simulink model "invertedPendolum"  (R2019b)
settings: Solver=VariableStepAuto  StartTime=0.0  StopTime=60  FixedStep=0.0001  RelTol=1e-4
InitFcn:
  | simulationVar
values from neighbouring files (symbols this model uses):
  tauMotMax = Ka * Id    (= 6208417600)    [simulationVar.m]
undefined symbols (not defined in the file or in its folder): smiData, X, Y, Z
libraries: sm_lib x29, simulink x6, nesl_utility x3
settings Model: Creator=alfyhack  LastModifiedBy=socci
settings SolverCC: AlgebraicLoopSolver=LineSearch
settings DebuggingCC: UnderSpecifiedDimensionMsg=warning
settings SFSimCC: CustomCodeUndefinedFunction=UseInterfaceOnly

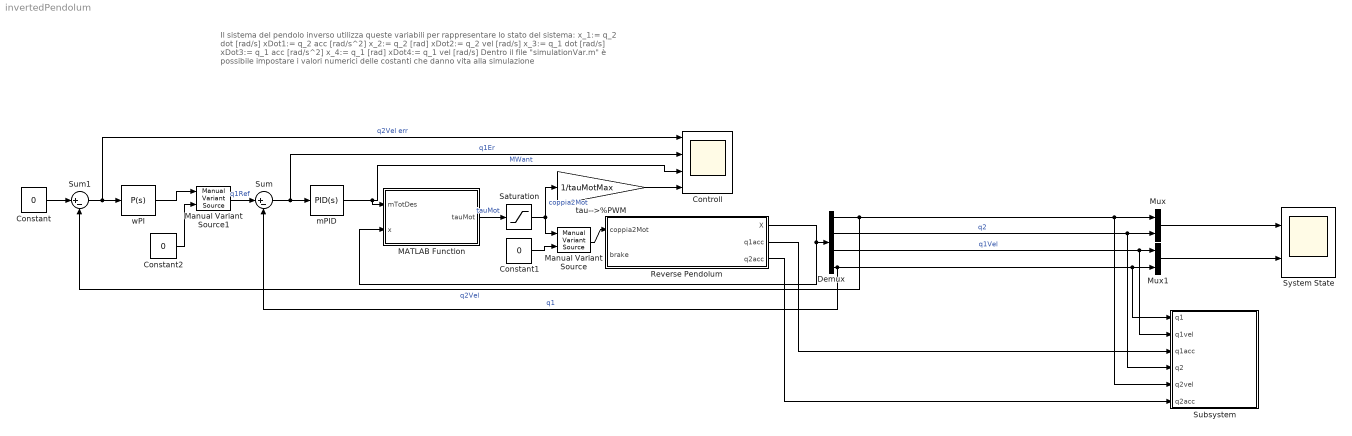
== system invertedPendolum ==
  note: Il sistema del pendolo inverso utilizza queste variabili per rappresentare lo stato del sistema:
      |
      | x_1:= q_2 dot  [rad/s]		xDot1:= q_2 acc   [rad/s^2]
      | x_2:= q_2        [rad]		xDot2:= q_2 vel    [rad/s]
      | x_3:= q_1 dot  [rad/s]		xDot3:= q_1 acc   [rad/s^2]
      | x_4:= q_1        [rad]		xDot4:= q_1 vel    [rad/s]
      |
      | Dentro il file "simulationVar.m" è possibile impostare i valori numerici delle costanti che danno vita alla simulazione
  Constant : Constant  Value=0
  Constant1 : Constant  Value=0
  Constant2 : Constant  Value=0
  Controll : Scope  NumInputPorts=4
  Demux : Demux
  MATLAB Function : MATLAB Function  TreatAsAtomicUnit=on
  Manual Variant Source : simulink/Signal Routing/Manual Variant Source  NumChoices=2  LabelModeActiveChoice=V_1
      settings: SourceProductName=Simulink
  Manual Variant Source1 : simulink/Signal Routing/Manual Variant Source  NumChoices=2  LabelModeActiveChoice=V_1
      settings: SourceProductName=Simulink
  Mux : Mux  Inputs=2
  Mux1 : Mux  Inputs=2
  Reverse Pendolum : Subsystem
  Saturation : Saturate  UpperLimit=tauMotMax  LowerLimit=-tauMotMax
  Subsystem : Subsystem
  Sum : Sum  Inputs=|+-
  Sum1 : Sum  Inputs=|+-
  System State : Scope  NumInputPorts=2
  mPID : simulink/Continuous/PID Controller  Controller=PID  Form=Parallel  TimeDomain=Continuous-time  SampleTime=-1  IntegratorMethod=Forward Euler  FilterMethod=Forward Euler  ControllerParametersSource=internal  P=44059890.2523914  I=6444277.98639226  D=74154463.3015082  UseFilter=on  N=34.9657186034109  TunerSelectOption=Transfer Function Based (PID Tuner App)  InitialConditionSource=internal  InitialConditionForIntegrator=0  InitialConditionForFilter=0  DifferentiatorICPrevScaledInput=0  ExternalReset=none  TrackingMode=off  Kt=1  LimitOutput=off  UpperSaturationLimit=1000  LowerSaturationLimit=1000  LinearizeAsGain=off  AntiWindupMode=none  Kb=1  POutMin=[]  POutMax=[]  IOutMin=[]  IOutMax=[]  DOutMin=[]  DOutMax=[]  NOutMin=[]  NOutMax=[]  SumOutMin=[]  SumOutMax=[]  SaturationOutMin=[]  SaturationOutMax=[]  PParamMin=[]  PParamMax=[]  IParamMin=[]  IParamMax=[]  DParamMin=[]  DParamMax=[]  NParamMin=[]  NParamMax=[]  KbParamMin=[]  KbParamMax=[]  KtParamMin=[]  KtParamMax=[]  KbOutMin=[]  KbOutMax=[]  KtOutMin=[]  KtOutMax=[]  IntegratorOutMin=[]  IntegratorOutMax=[]  FilterOutMin=[]  FilterOutMax=[]  SumI1OutMin=[]  SumI1OutMax=[]  SumI2OutMin=[]  SumI2OutMax=[]  SumI3OutMin=[]  SumI3OutMax=[]  SumI4OutMin=[]  SumI4OutMax=[]  SumDOutMin=[]  SumDOutMax=[]  DifferentiatorOutMin=[]  DifferentiatorOutMax=[]  FilterDiffOutCoefMin=[]  FilterDiffOutCoefMax=[]  ReciprocalOutMin=[]  ReciprocalOutMax=[]  SumDenOutMin=[]  SumDenOutMax=[]  SumNumOutMin=[]  SumNumOutMax=[]  DivideOutMin=[]  DivideOutMax=[]  IntegratorContinuousStateAttributes=''  IntegratorStateMustResolveToSignalObject=off  IntegratorRTWStateStorageClass=Auto  FilterContinuousStateAttributes=''  FilterStateMustResolveToSignalObject=off  FilterRTWStateStorageClass=Auto  ParallelPVariant=InternalParameters  IdealPVariant=Disabled  IVariant=InternalParameters  DVariant=InternalParameters  IntegratorVariant=Continuous  SatVariant=Disabled  AWVariant=Passthrough  PCopyVariant=Disabled  TRVariant=Disabled  FdbkBlocksVariant=Forward  IdealPFdbkVariant=Disabled  SatFdbkVariant=Disabled  DerivativeFilterVariant=ContFilter  NVariant=InternalParameters  NCopyVariant=Disabled  FilterICVariant=InternalICsFilter  IntegratorICVariant=InternalICs  ExternalResetVariant=Disabled  TRSumVariant=Passthrough  SumFdbkVariant=Disabled  SumVariant=Sum_PID
  tau-->%PWM : Gain  Gain=1/tauMotMax
  wPI : simulink/Continuous/PID Controller  Controller=P  Form=Parallel  TimeDomain=Continuous-time  SampleTime=-1  IntegratorMethod=Forward Euler  FilterMethod=Forward Euler  ControllerParametersSource=internal  P=0.000273498312206375  I=0.001  D=1  UseFilter=on  N=2000  TunerSelectOption=Transfer Function Based (PID Tuner App)  InitialConditionSource=internal  InitialConditionForIntegrator=0  InitialConditionForFilter=0  DifferentiatorICPrevScaledInput=0  ExternalReset=none  TrackingMode=off  Kt=1  LimitOutput=on  UpperSaturationLimit=0.1  LowerSaturationLimit=-0.1  LinearizeAsGain=off  AntiWindupMode=none  Kb=1  POutMin=[]  POutMax=[]  IOutMin=[]  IOutMax=[]  DOutMin=[]  DOutMax=[]  NOutMin=[]  NOutMax=[]  SumOutMin=[]  SumOutMax=[]  SaturationOutMin=[]  SaturationOutMax=[]  PParamMin=[]  PParamMax=[]  IParamMin=[]  IParamMax=[]  DParamMin=[]  DParamMax=[]  NParamMin=[]  NParamMax=[]  KbParamMin=[]  KbParamMax=[]  KtParamMin=[]  KtParamMax=[]  KbOutMin=[]  KbOutMax=[]  KtOutMin=[]  KtOutMax=[]  IntegratorOutMin=[]  IntegratorOutMax=[]  FilterOutMin=[]  FilterOutMax=[]  SumI1OutMin=[]  SumI1OutMax=[]  SumI2OutMin=[]  SumI2OutMax=[]  SumI3OutMin=[]  SumI3OutMax=[]  SumI4OutMin=[]  SumI4OutMax=[]  SumDOutMin=[]  SumDOutMax=[]  DifferentiatorOutMin=[]  DifferentiatorOutMax=[]  FilterDiffOutCoefMin=[]  FilterDiffOutCoefMax=[]  ReciprocalOutMin=[]  ReciprocalOutMax=[]  SumDenOutMin=[]  SumDenOutMax=[]  SumNumOutMin=[]  SumNumOutMax=[]  DivideOutMin=[]  DivideOutMax=[]  IntegratorContinuousStateAttributes=''  IntegratorStateMustResolveToSignalObject=off  IntegratorRTWStateStorageClass=Auto  FilterContinuousStateAttributes=''  FilterStateMustResolveToSignalObject=off  FilterRTWStateStorageClass=Auto  ParallelPVariant=InternalParameters  IdealPVariant=Disabled  IVariant=Disabled  DVariant=Disabled  IntegratorVariant=Disabled  SatVariant=Enabled  AWVariant=Disabled  PCopyVariant=Disabled  TRVariant=Disabled  FdbkBlocksVariant=Forward  IdealPFdbkVariant=Disabled  SatFdbkVariant=Disabled  DerivativeFilterVariant=Disabled  NVariant=Disabled  NCopyVariant=Disabled_SignalSpec  FilterICVariant=Disabled  IntegratorICVariant=Disabled  ExternalResetVariant=Disabled  TRSumVariant=Passthrough  SumFdbkVariant=Disabled  SumVariant=Passthrough_P
  wires:
  Demux/4 -> Subsystem/1(q1), Mux1/2, Sum/2  "q1"
  Demux/1 -> Subsystem/5(q2vel), Mux/1, Sum1/2  "q2Vel"
  MATLAB Function/1(tauMot) -> Saturation/1  "tauMot"
  mPID/1 -> Controll/3, MATLAB Function/1(mTotDes)  "MWant"
  Sum/1 -> Controll/2, mPID/1  "q1Er"
  wPI/1 -> Manual Variant Source1/1
  Constant/1 -> Sum1/1
  Sum1/1 -> Controll/1, wPI/1  "q2Vel err"
  Saturation/1 -> tau-->%PWM/1, Manual Variant Source/1  "coppia2Mot"
  Reverse Pendolum/1(X) -> Demux/1, MATLAB Function/2(x)
  Demux/3 -> Subsystem/2(q1vel), Mux1/1  "q1Vel"
  Mux1/1 -> System State/2
  Mux/1 -> System State/1
  tau-->%PWM/1 -> Controll/4
  Manual Variant Source/1 -> Reverse Pendolum/1(coppia2Mot)
  Constant1/1 -> Manual Variant Source/2
  Manual Variant Source1/1 -> Sum/1  "q1Ref"
  Constant2/1 -> Manual Variant Source1/2
  Reverse Pendolum/2(q1acc) -> Subsystem/3(q1acc)
  Reverse Pendolum/3(q2acc) -> Subsystem/6(q2acc)
  Demux/2 -> Subsystem/4(q2), Mux/2  "q2"

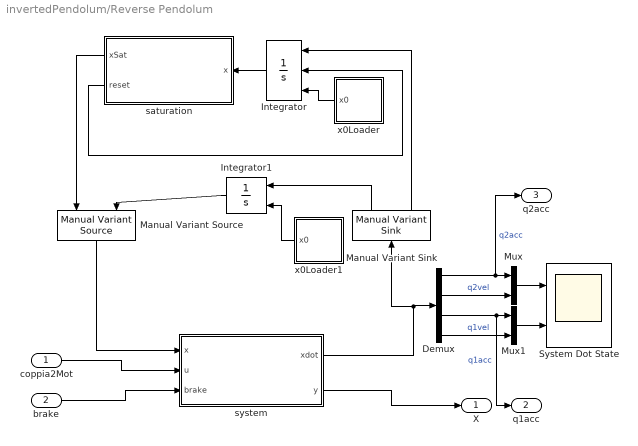
== system invertedPendolum/Reverse Pendolum ==
  coppia2Mot : Inport
  brake : Inport  Port=2
  Demux : Demux
  Integrator : Integrator  ExternalReset=rising  InitialConditionSource=external  InitialCondition=[0,0.1,0]
  Integrator1 : Integrator  InitialConditionSource=external
  Manual Variant Sink : simulink/Signal Routing/Manual Variant Sink  NumChoices=2  LabelModeActiveChoice=V_2
      settings: SourceProductName=Simulink
  Manual Variant Source : simulink/Signal Routing/Manual Variant Source  NumChoices=2  LabelModeActiveChoice=V_1
      settings: SourceProductName=Simulink
  Mux : Mux  Inputs=2
  Mux1 : Mux  Inputs=2
  System Dot State : Scope  NumInputPorts=2
  saturation : MATLAB Function  TreatAsAtomicUnit=on
  system : MATLAB Function  TreatAsAtomicUnit=on
  x0Loader : MATLAB Function  TreatAsAtomicUnit=on
  x0Loader1 : MATLAB Function  TreatAsAtomicUnit=on
  X : Outport  VectorParamsAs1DForOutWhenUnconnected=off
  q1acc : Outport  Port=2  VectorParamsAs1DForOutWhenUnconnected=off
  q2acc : Outport  Port=3  VectorParamsAs1DForOutWhenUnconnected=off
  wires:
  x0Loader/1(x0) -> Integrator/3
  Integrator/1 -> saturation/1(x)
  saturation/2(reset) -> Integrator/2
  coppia2Mot/1 -> system/2(u)
  system/2(y) -> X/1
  Mux/1 -> System Dot State/1
  Demux/3 -> q1acc/1, Mux1/1  "q1acc"
  Demux/1 -> q2acc/1, Mux/1  "q2acc"
  system/1(xdot) -> Manual Variant Sink/1, Demux/1
  Demux/2 -> Mux/2  "q2vel"
  Demux/4 -> Mux1/2  "q1vel"
  Mux1/1 -> System Dot State/2
  Manual Variant Sink/2 -> Integrator/1
  saturation/1(xSat) -> Manual Variant Source/1
  Integrator1/1 -> Manual Variant Source/2
  Manual Variant Sink/1 -> Integrator1/1
  Manual Variant Source/1 -> system/1(x)
  x0Loader1/1(x0) -> Integrator1/2
  brake/1 -> system/3(brake)

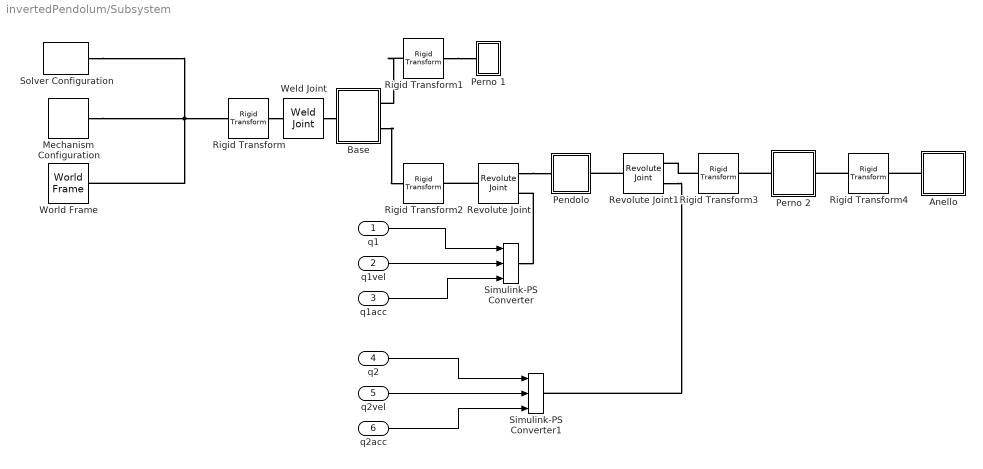
== system invertedPendolum/Subsystem ==
  q1 : Inport
  q1vel : Inport  Port=2
  q1acc : Inport  Port=3
  q2 : Inport  Port=4
  q2vel : Inport  Port=5
  q2acc : Inport  Port=6
  "Anello " : Subsystem
  Base : Subsystem
  Mechanism Configuration : sm_lib/Utilities/Mechanism Configuration  UniformGravity=Constant  GravityVector=[0 0 0]  GravityUnits=m/s^2  LinearizationDelta=0.001
  Pendolo : Subsystem
  Perno 1 : Subsystem
  Perno 2 : Subsystem
  Revolute Joint : sm_lib/Joints/Revolute Joint  JointMode=Normal  SenseConstraintForce=off  SenseConstraintForceX=off  SenseConstraintForceY=off  SenseConstraintForceZ=off  SenseConstraintTorque=off  SenseConstraintTorqueX=off  SenseConstraintTorqueY=off  SenseConstraintTorqueZ=off  SenseTotalForce=off  SenseTotalForceX=off  SenseTotalForceY=off  SenseTotalForceZ=off  SenseTotalTorque=off  SenseTotalTorqueX=off  SenseTotalTorqueY=off  SenseTotalTorqueZ=off  CompositeWrenchDir=FollowerOnBase  CompositeWrenchFrame=BaseFrame  EquilibriumPosition=0  EquilibriumPositionUnits=deg  SpringStiffness=0  SpringStiffnessUnits=N*m/deg  DampingCoefficient=0  DampingCoefficientUnits=N*m/(deg/s)  TorqueActuationMode=ComputedTorque  MotionActuationMode=InputMotion  SensePosition=off  SenseVelocity=off  SenseAcceleration=off  SenseTorqueForce=off  SenseLowerLimitTorqueForce=off  SenseUpperLimitTorqueForce=off  LowerLimitSpecify=off  LowerLimitBound=-90  LowerLimitBoundUnits=deg  LowerLimitStiffness=1e4  LowerLimitStiffnessUnits=N*m/deg  LowerLimitDamping=10  LowerLimitDampingUnits=N*m/(deg/s)  LowerLimitTransitionRegionWidth=0.1  LowerLimitTransitionRegionWidthUnits=deg  UpperLimitSpecify=off  UpperLimitBound=90  UpperLimitBoundUnits=deg  UpperLimitStiffness=1e4  UpperLimitStiffnessUnits=N*m/deg  UpperLimitDamping=10  UpperLimitDampingUnits=N*m/(deg/s)  UpperLimitTransitionRegionWidth=0.1  UpperLimitTransitionRegionWidthUnits=deg  PositionTargetSpecify=on  PositionTargetPriority=Low  PositionTargetValue=smiData.RevoluteJoint(2).Rz.Pos  PositionTargetValueUnits=deg  VelocityTargetSpecify=off  VelocityTargetPriority=High  VelocityTargetValue=0  VelocityTargetValueUnits=deg/s
  Revolute Joint1 : sm_lib/Joints/Revolute Joint  JointMode=Normal  SenseConstraintForce=off  SenseConstraintForceX=off  SenseConstraintForceY=off  SenseConstraintForceZ=off  SenseConstraintTorque=off  SenseConstraintTorqueX=off  SenseConstraintTorqueY=off  SenseConstraintTorqueZ=off  SenseTotalForce=off  SenseTotalForceX=off  SenseTotalForceY=off  SenseTotalForceZ=off  SenseTotalTorque=off  SenseTotalTorqueX=off  SenseTotalTorqueY=off  SenseTotalTorqueZ=off  CompositeWrenchDir=FollowerOnBase  CompositeWrenchFrame=BaseFrame  EquilibriumPosition=0  EquilibriumPositionUnits=deg  SpringStiffness=0  SpringStiffnessUnits=N*m/deg  DampingCoefficient=0  DampingCoefficientUnits=N*m/(deg/s)  TorqueActuationMode=ComputedTorque  MotionActuationMode=InputMotion  SensePosition=off  SenseVelocity=off  SenseAcceleration=off  SenseTorqueForce=off  SenseLowerLimitTorqueForce=off  SenseUpperLimitTorqueForce=off  LowerLimitSpecify=off  LowerLimitBound=-90  LowerLimitBoundUnits=deg  LowerLimitStiffness=1e4  LowerLimitStiffnessUnits=N*m/deg  LowerLimitDamping=10  LowerLimitDampingUnits=N*m/(deg/s)  LowerLimitTransitionRegionWidth=0.1  LowerLimitTransitionRegionWidthUnits=deg  UpperLimitSpecify=off  UpperLimitBound=90  UpperLimitBoundUnits=deg  UpperLimitStiffness=1e4  UpperLimitStiffnessUnits=N*m/deg  UpperLimitDamping=10  UpperLimitDampingUnits=N*m/(deg/s)  UpperLimitTransitionRegionWidth=0.1  UpperLimitTransitionRegionWidthUnits=deg  PositionTargetSpecify=off  PositionTargetPriority=High  PositionTargetValue=0  PositionTargetValueUnits=deg  VelocityTargetSpecify=off  VelocityTargetPriority=High  VelocityTargetValue=0  VelocityTargetValueUnits=deg/s
  Rigid Transform{,1,3..4} (4 alike) : sm_lib/Frames and Transforms/Rigid Transform  TranslationMethod=None  TranslationStandardOffset=0  TranslationLengthUnit=m  TranslationStandardAxis=+Z  TranslationCartesianOffset=[0 0 0]  TranslationROffset=0  TranslationROffsetUnits=m  TranslationZOffset=0  TranslationZOffsetUnits=m  TranslationThetaOffset=0  TranslationThetaOffsetUnits=deg  RotationMethod=None  RotationAngleUnits=deg  RotationStandardAxis=+Z  RotationAngle=0.0  RotationArbitraryAxis=[0 0 1]  FollAlignAxisA=+X  BaseAlignAxisA=+Y  FollAlignAxisB=+Y  BaseAlignAxisB=+Z  RotationSequenceAxes=FollowerAxes  RotationSequence=XYX  RotationSequenceAngles=[0 0 0]  RotationSequenceAnglesUnits=deg  RotationMatrix=[1 0 0; 0 1 0; 0 0 1]
  Rigid Transform2 : sm_lib/Frames and Transforms/Rigid Transform  TranslationMethod=None  TranslationStandardOffset=0  TranslationLengthUnit=m  TranslationStandardAxis=+Z  TranslationCartesianOffset=[0 0 0]  TranslationROffset=0  TranslationROffsetUnits=m  TranslationZOffset=0  TranslationZOffsetUnits=m  TranslationThetaOffset=0  TranslationThetaOffsetUnits=deg  RotationMethod=RotationSequence  RotationAngleUnits=deg  RotationStandardAxis=+Z  RotationAngle=0.0  RotationArbitraryAxis=[0 0 1]  FollAlignAxisA=+X  BaseAlignAxisA=+Y  FollAlignAxisB=+Y  BaseAlignAxisB=+Z  RotationSequenceAxes=FollowerAxes  RotationSequence=XYZ  RotationSequenceAngles=[0 0 90 ]  RotationSequenceAnglesUnits=deg  RotationMatrix=[1 0 0; 0 1 0; 0 0 1]
  Simulink-PS Converter : nesl_utility/Simulink-PS Converter  PhysicalDomain=network_engine_domain  SubClassName=ps_input  LeftPortType=input  RightPortType=output  PseudoPeriodic=off  Frequencies=[]  NoiseDistribution=none  NoiseParameters=[]  Unit=1  AffineConversion=off  FilteringAndDerivatives=provide  SimscapeFilterOrder=1  InputFilterTimeConstant=0.001  UdotUserProvided=2
  Simulink-PS Converter1 : nesl_utility/Simulink-PS Converter  PhysicalDomain=network_engine_domain  SubClassName=ps_input  LeftPortType=input  RightPortType=output  PseudoPeriodic=off  Frequencies=[]  NoiseDistribution=none  NoiseParameters=[]  Unit=1  AffineConversion=off  FilteringAndDerivatives=provide  SimscapeFilterOrder=1  InputFilterTimeConstant=0.001  UdotUserProvided=2
  Solver Configuration : nesl_utility/Solver Configuration  PhysicalDomain=network_engine_domain  SubClassName=solver  LeftPortType=input  RightPortType=generic  Tones=[]  Harmonics=[]  SimulateNoise=off  Profile=off  UseLocalSampling=off  EnableSwitchedLinearOptims=on  FrequencyDomain=off  UseCCode=off  RelTol=0.001  AbsTol=1e-06  MinStep=1e-09  ToWorkspace=off  RevertToSquareIcSolve=off  NumHomotopyIterations=100  PhasorMode=off  PhasorModeNumHarmonics=1  DoDC=off  ResidualTolerance=1e-09  UseLocalSolver=off  LocalSolverChoice=NE_BACKWARD_EULER_ADVANCER  LocalSolverSampleTime=0.001  DoFixedCost=off  MaxNonlinIter=3  MaxModeIter=2  LinearAlgebra=auto  EquationFormulation=NE_TIME_EF  DelaysMemoryBudget=1024  AutomaticFiltering=on  FilteringTimeConstant=0.001  PartitionStorageMethod=AS_NEEDED  PartitionMemoryBudget=1024  PartitionMethod=ROBUST
  Weld Joint : sm_lib/Joints/Weld Joint  JointMode=Normal  SenseConstraintForce=off  SenseConstraintForceX=off  SenseConstraintForceY=off  SenseConstraintForceZ=off  SenseConstraintTorque=off  SenseConstraintTorqueX=off  SenseConstraintTorqueY=off  SenseConstraintTorqueZ=off  SenseTotalForce=off  SenseTotalForceX=off  SenseTotalForceY=off  SenseTotalForceZ=off  SenseTotalTorque=off  SenseTotalTorqueX=off  SenseTotalTorqueY=off  SenseTotalTorqueZ=off  CompositeWrenchDir=FollowerOnBase  CompositeWrenchFrame=BaseFrame
  World Frame : sm_lib/Frames and Transforms/World Frame
  wires:
  q1/1 -> Simulink-PS Converter/1
  q1vel/1 -> Simulink-PS Converter/2
  q1acc/1 -> Simulink-PS Converter/3
  q2acc/1 -> Simulink-PS Converter1/3
  q2/1 -> Simulink-PS Converter1/1
  q2vel/1 -> Simulink-PS Converter1/2
  connections:
  Solver Configuration/RConn1 -- World Frame/RConn1 -- Rigid Transform/LConn1 -- Mechanism Configuration/RConn1
  Rigid Transform/RConn1 -- Weld Joint/LConn1
  Weld Joint/RConn1 -- Base/LConn1
  Rigid Transform1/LConn1 -- Base/RConn1
  Rigid Transform1/RConn1 -- Perno 1/LConn1
  Base/RConn2 -- Rigid Transform2/LConn1
  Revolute Joint/RConn1 -- Rigid Transform2/RConn1
  Simulink-PS Converter/RConn1 -- Revolute Joint/LConn2
  Revolute Joint/LConn1 -- Pendolo/LConn1
  Revolute Joint1/RConn1 -- Pendolo/RConn1
  Rigid Transform3/RConn1 -- Revolute Joint1/LConn1
  Perno 2/LConn1 -- Rigid Transform3/LConn1
  Rigid Transform4/LConn1 -- Perno 2/RConn1
  "Anello "/LConn1 -- Rigid Transform4/RConn1
  Revolute Joint1/LConn2 -- Simulink-PS Converter1/RConn1

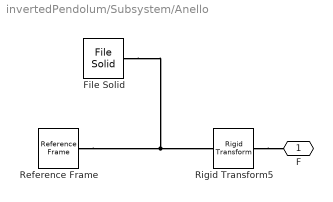
== system invertedPendolum/Subsystem/Anello  ==
  File Solid : sm_lib/Body Elements/File Solid  ExtGeomFileName=Anello_ipt_98140efb.STEP  UnitType=FromFile  ExtGeomFileUnits=m  StepReaderType=HEX  ExportEntireGeometry=off  InertiaType=Custom  Mass=smiData.Solid(4).mass  MassUnits=kg  CenterOfMass=smiData.Solid(4).CoM  CenterOfMassUnits=mm  MomentsOfInertia=smiData.Solid(4).MoI  MomentsOfInertiaUnits=kg*mm^2  ProductsOfInertia=smiData.Solid(4).PoI  ProductsOfInertiaUnits=kg*mm^2  BasedOnType=DensityFromFile  Density=1000  DensityUnits=kg/m^3  DoExposeReferenceFrame=on  SerializedFrames=<Frames/>  GraphicType=FromGeometry  MarkerShape=Sphere  MarkerSize=10  GraphicVisPropType=SimpleVisualProperties  GraphicDiffuseColor=[0.8 1.0 0.2]  GraphicSpecularColor=[0.5 0.5 0.5 1.0]  GraphicAmbientColor=[0.15 0.15 0.15 1.0]  GraphicEmissiveColor=[0.0 0.0 0.0 1.0]  GraphicShininess=75  GraphicOpacity=1.0
  Reference Frame : sm_lib/Frames and Transforms/Reference Frame
  Rigid Transform5 : sm_lib/Frames and Transforms/Rigid Transform  TranslationMethod=Cartesian  TranslationStandardOffset=0  TranslationLengthUnit=mm  TranslationStandardAxis=+Z  TranslationCartesianOffset=smiData.RigidTransform(9).translation  TranslationROffset=0  TranslationROffsetUnits=m  TranslationZOffset=0  TranslationZOffsetUnits=m  TranslationThetaOffset=0  TranslationThetaOffsetUnits=deg  RotationMethod=ArbitraryAxis  RotationAngleUnits=rad  RotationStandardAxis=+Z  RotationAngle=smiData.RigidTransform(9).angle  RotationArbitraryAxis=smiData.RigidTransform(9).axis  FollAlignAxisA=+X  BaseAlignAxisA=+Y  FollAlignAxisB=+Y  BaseAlignAxisB=+Z  RotationSequenceAxes=FollowerAxes  RotationSequence=XYX  RotationSequenceAngles=[0 0 0]  RotationSequenceAnglesUnits=deg  RotationMatrix=[1 0 0; 0 1 0; 0 0 1]
  F : PMIOPort  Side=Left
  connections:
  Reference Frame/RConn1 -- File Solid/RConn1 -- Rigid Transform5/LConn1
  Rigid Transform5/RConn1 -- F/RConn1

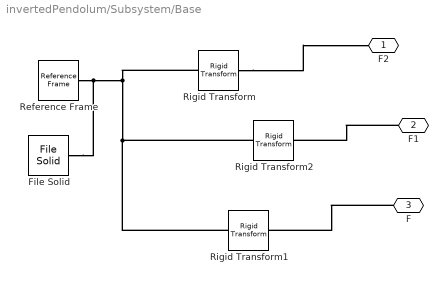
== system invertedPendolum/Subsystem/Base ==
  File Solid : sm_lib/Body Elements/File Solid  ExtGeomFileName=Base_ipt_2f93e7fb.STEP  UnitType=FromFile  ExtGeomFileUnits=m  StepReaderType=HEX  ExportEntireGeometry=off  InertiaType=Custom  Mass=smiData.Solid(1).mass  MassUnits=kg  CenterOfMass=smiData.Solid(1).CoM  CenterOfMassUnits=mm  MomentsOfInertia=smiData.Solid(1).MoI  MomentsOfInertiaUnits=kg*mm^2  ProductsOfInertia=smiData.Solid(1).PoI  ProductsOfInertiaUnits=kg*mm^2  BasedOnType=DensityFromFile  Density=1000  DensityUnits=kg/m^3  DoExposeReferenceFrame=on  SerializedFrames=<Frames/>  GraphicType=FromGeometry  MarkerShape=Sphere  MarkerSize=10  GraphicVisPropType=SimpleVisualProperties  GraphicDiffuseColor=[0.2 0.2 1.0]  GraphicSpecularColor=[0.5 0.5 0.5 1.0]  GraphicAmbientColor=[0.15 0.15 0.15 1.0]  GraphicEmissiveColor=[0.0 0.0 0.0 1.0]  GraphicShininess=75  GraphicOpacity=1.0
  Reference Frame : sm_lib/Frames and Transforms/Reference Frame
  Rigid Transform : sm_lib/Frames and Transforms/Rigid Transform  TranslationMethod=Cartesian  TranslationStandardOffset=0  TranslationLengthUnit=mm  TranslationStandardAxis=+Z  TranslationCartesianOffset=smiData.RigidTransform(6).translation  TranslationROffset=0  TranslationROffsetUnits=m  TranslationZOffset=0  TranslationZOffsetUnits=m  TranslationThetaOffset=0  TranslationThetaOffsetUnits=deg  RotationMethod=ArbitraryAxis  RotationAngleUnits=rad  RotationStandardAxis=+Z  RotationAngle=smiData.RigidTransform(6).angle  RotationArbitraryAxis=smiData.RigidTransform(6).axis  FollAlignAxisA=+X  BaseAlignAxisA=+Y  FollAlignAxisB=+Y  BaseAlignAxisB=+Z  RotationSequenceAxes=FollowerAxes  RotationSequence=XYX  RotationSequenceAngles=[0 0 0]  RotationSequenceAnglesUnits=deg  RotationMatrix=[1 0 0; 0 1 0; 0 0 1]
  Rigid Transform1 : sm_lib/Frames and Transforms/Rigid Transform  TranslationMethod=Cartesian  TranslationStandardOffset=0  TranslationLengthUnit=mm  TranslationStandardAxis=+Z  TranslationCartesianOffset=smiData.RigidTransform(1).translation  TranslationROffset=0  TranslationROffsetUnits=m  TranslationZOffset=0  TranslationZOffsetUnits=m  TranslationThetaOffset=0  TranslationThetaOffsetUnits=deg  RotationMethod=ArbitraryAxis  RotationAngleUnits=rad  RotationStandardAxis=+Z  RotationAngle=smiData.RigidTransform(1).angle  RotationArbitraryAxis=smiData.RigidTransform(1).axis  FollAlignAxisA=+X  BaseAlignAxisA=+Y  FollAlignAxisB=+Y  BaseAlignAxisB=+Z  RotationSequenceAxes=FollowerAxes  RotationSequence=XYX  RotationSequenceAngles=[0 0 0]  RotationSequenceAnglesUnits=deg  RotationMatrix=[1 0 0; 0 1 0; 0 0 1]
  Rigid Transform2 : sm_lib/Frames and Transforms/Rigid Transform  TranslationMethod=Cartesian  TranslationStandardOffset=0  TranslationLengthUnit=mm  TranslationStandardAxis=+Z  TranslationCartesianOffset=smiData.RigidTransform(4).translation  TranslationROffset=0  TranslationROffsetUnits=m  TranslationZOffset=0  TranslationZOffsetUnits=m  TranslationThetaOffset=0  TranslationThetaOffsetUnits=deg  RotationMethod=ArbitraryAxis  RotationAngleUnits=rad  RotationStandardAxis=+Z  RotationAngle=smiData.RigidTransform(4).angle  RotationArbitraryAxis=smiData.RigidTransform(4).axis  FollAlignAxisA=+X  BaseAlignAxisA=+Y  FollAlignAxisB=+Y  BaseAlignAxisB=+Z  RotationSequenceAxes=FollowerAxes  RotationSequence=XYX  RotationSequenceAngles=[0 0 0]  RotationSequenceAnglesUnits=deg  RotationMatrix=[1 0 0; 0 1 0; 0 0 1]
  F2 : PMIOPort  Side=Right
  F1 : PMIOPort  Port=2  Side=Right
  F : PMIOPort  Port=3  Side=Left
  connections:
  Reference Frame/RConn1 -- File Solid/RConn1 -- Rigid Transform1/LConn1 -- Rigid Transform2/LConn1 -- Rigid Transform/LConn1
  Rigid Transform/RConn1 -- F2/RConn1
  F1/RConn1 -- Rigid Transform2/RConn1
  F/RConn1 -- Rigid Transform1/RConn1

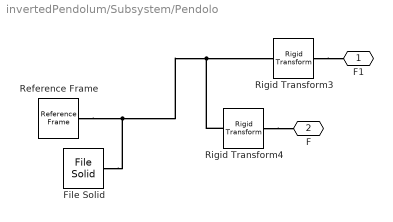
== system invertedPendolum/Subsystem/Pendolo ==
  File Solid : sm_lib/Body Elements/File Solid  ExtGeomFileName=Pendolo_ipt_9bec4f24.STEP  UnitType=FromFile  ExtGeomFileUnits=m  StepReaderType=HEX  ExportEntireGeometry=off  InertiaType=Custom  Mass=smiData.Solid(3).mass  MassUnits=kg  CenterOfMass=smiData.Solid(3).CoM  CenterOfMassUnits=mm  MomentsOfInertia=smiData.Solid(3).MoI  MomentsOfInertiaUnits=kg*mm^2  ProductsOfInertia=smiData.Solid(3).PoI  ProductsOfInertiaUnits=kg*mm^2  BasedOnType=DensityFromFile  Density=1000  DensityUnits=kg/m^3  DoExposeReferenceFrame=on  SerializedFrames=<Frames/>  GraphicType=FromGeometry  MarkerShape=Sphere  MarkerSize=10  GraphicVisPropType=SimpleVisualProperties  GraphicDiffuseColor=[0.8 1.0 0.2]  GraphicSpecularColor=[0.5 0.5 0.5 1.0]  GraphicAmbientColor=[0.15 0.15 0.15 1.0]  GraphicEmissiveColor=[0.0 0.0 0.0 1.0]  GraphicShininess=75  GraphicOpacity=1.0
  Reference Frame : sm_lib/Frames and Transforms/Reference Frame
  Rigid Transform3 : sm_lib/Frames and Transforms/Rigid Transform  TranslationMethod=Cartesian  TranslationStandardOffset=0  TranslationLengthUnit=mm  TranslationStandardAxis=+Z  TranslationCartesianOffset=smiData.RigidTransform(8).translation  TranslationROffset=0  TranslationROffsetUnits=m  TranslationZOffset=0  TranslationZOffsetUnits=m  TranslationThetaOffset=0  TranslationThetaOffsetUnits=deg  RotationMethod=ArbitraryAxis  RotationAngleUnits=rad  RotationStandardAxis=+Z  RotationAngle=smiData.RigidTransform(8).angle  RotationArbitraryAxis=smiData.RigidTransform(8).axis  FollAlignAxisA=+X  BaseAlignAxisA=+Y  FollAlignAxisB=+Y  BaseAlignAxisB=+Z  RotationSequenceAxes=FollowerAxes  RotationSequence=XYX  RotationSequenceAngles=[0 0 0]  RotationSequenceAnglesUnits=deg  RotationMatrix=[1 0 0; 0 1 0; 0 0 1]
  Rigid Transform4 : sm_lib/Frames and Transforms/Rigid Transform  TranslationMethod=Cartesian  TranslationStandardOffset=0  TranslationLengthUnit=mm  TranslationStandardAxis=+Z  TranslationCartesianOffset=smiData.RigidTransform(3).translation  TranslationROffset=0  TranslationROffsetUnits=m  TranslationZOffset=0  TranslationZOffsetUnits=m  TranslationThetaOffset=0  TranslationThetaOffsetUnits=deg  RotationMethod=ArbitraryAxis  RotationAngleUnits=rad  RotationStandardAxis=+Z  RotationAngle=smiData.RigidTransform(3).angle  RotationArbitraryAxis=smiData.RigidTransform(3).axis  FollAlignAxisA=+X  BaseAlignAxisA=+Y  FollAlignAxisB=+Y  BaseAlignAxisB=+Z  RotationSequenceAxes=FollowerAxes  RotationSequence=XYX  RotationSequenceAngles=[0 0 0]  RotationSequenceAnglesUnits=deg  RotationMatrix=[1 0 0; 0 1 0; 0 0 1]
  F1 : PMIOPort  Side=Right
  "F " : PMIOPort  Port=2  Side=Left
  connections:
  Reference Frame/RConn1 -- File Solid/RConn1 -- Rigid Transform4/LConn1 -- Rigid Transform3/LConn1
  Rigid Transform3/RConn1 -- F1/RConn1
  Rigid Transform4/RConn1 -- "F "/RConn1

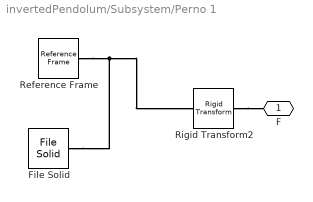
== system invertedPendolum/Subsystem/Perno 1 ==
  File Solid : sm_lib/Body Elements/File Solid  ExtGeomFileName=Perno_ipt_13122ac9.STEP  UnitType=FromFile  ExtGeomFileUnits=m  StepReaderType=HEX  ExportEntireGeometry=off  InertiaType=Custom  Mass=smiData.Solid(2).mass  MassUnits=kg  CenterOfMass=smiData.Solid(2).CoM  CenterOfMassUnits=mm  MomentsOfInertia=smiData.Solid(2).MoI  MomentsOfInertiaUnits=kg*mm^2  ProductsOfInertia=smiData.Solid(2).PoI  ProductsOfInertiaUnits=kg*mm^2  BasedOnType=DensityFromFile  Density=1000  DensityUnits=kg/m^3  DoExposeReferenceFrame=on  SerializedFrames=<Frames/>  GraphicType=FromGeometry  MarkerShape=Sphere  MarkerSize=10  GraphicVisPropType=SimpleVisualProperties  GraphicDiffuseColor=[0.8 0.8 0.8]  GraphicSpecularColor=[0.5 0.5 0.5 1.0]  GraphicAmbientColor=[0.15 0.15 0.15 1.0]  GraphicEmissiveColor=[0.0 0.0 0.0 1.0]  GraphicShininess=75  GraphicOpacity=1.0
  Reference Frame : sm_lib/Frames and Transforms/Reference Frame
  Rigid Transform2 : sm_lib/Frames and Transforms/Rigid Transform  TranslationMethod=Cartesian  TranslationStandardOffset=0  TranslationLengthUnit=mm  TranslationStandardAxis=+Z  TranslationCartesianOffset=smiData.RigidTransform(5).translation  TranslationROffset=0  TranslationROffsetUnits=m  TranslationZOffset=0  TranslationZOffsetUnits=m  TranslationThetaOffset=0  TranslationThetaOffsetUnits=deg  RotationMethod=ArbitraryAxis  RotationAngleUnits=rad  RotationStandardAxis=+Z  RotationAngle=smiData.RigidTransform(5).angle  RotationArbitraryAxis=smiData.RigidTransform(5).axis  FollAlignAxisA=+X  BaseAlignAxisA=+Y  FollAlignAxisB=+Y  BaseAlignAxisB=+Z  RotationSequenceAxes=FollowerAxes  RotationSequence=XYX  RotationSequenceAngles=[0 0 0]  RotationSequenceAnglesUnits=deg  RotationMatrix=[1 0 0; 0 1 0; 0 0 1]
  F : PMIOPort  Side=Left
  connections:
  Reference Frame/RConn1 -- File Solid/RConn1 -- Rigid Transform2/LConn1
  Rigid Transform2/RConn1 -- F/RConn1

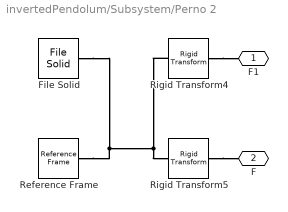
== system invertedPendolum/Subsystem/Perno 2 ==
  File Solid : sm_lib/Body Elements/File Solid  ExtGeomFileName=Perno_ipt_13122ac9.STEP  UnitType=FromFile  ExtGeomFileUnits=m  StepReaderType=HEX  ExportEntireGeometry=off  InertiaType=Custom  Mass=smiData.Solid(2).mass  MassUnits=kg  CenterOfMass=smiData.Solid(2).CoM  CenterOfMassUnits=mm  MomentsOfInertia=smiData.Solid(2).MoI  MomentsOfInertiaUnits=kg*mm^2  ProductsOfInertia=smiData.Solid(2).PoI  ProductsOfInertiaUnits=kg*mm^2  BasedOnType=DensityFromFile  Density=1000  DensityUnits=kg/m^3  DoExposeReferenceFrame=on  SerializedFrames=<Frames/>  GraphicType=FromGeometry  MarkerShape=Sphere  MarkerSize=10  GraphicVisPropType=SimpleVisualProperties  GraphicDiffuseColor=[0.8 0.8 0.8]  GraphicSpecularColor=[0.5 0.5 0.5 1.0]  GraphicAmbientColor=[0.15 0.15 0.15 1.0]  GraphicEmissiveColor=[0.0 0.0 0.0 1.0]  GraphicShininess=75  GraphicOpacity=1.0
  Reference Frame : sm_lib/Frames and Transforms/Reference Frame
  Rigid Transform4 : sm_lib/Frames and Transforms/Rigid Transform  TranslationMethod=Cartesian  TranslationStandardOffset=0  TranslationLengthUnit=mm  TranslationStandardAxis=+Z  TranslationCartesianOffset=smiData.RigidTransform(10).translation  TranslationROffset=0  TranslationROffsetUnits=m  TranslationZOffset=0  TranslationZOffsetUnits=m  TranslationThetaOffset=0  TranslationThetaOffsetUnits=deg  RotationMethod=ArbitraryAxis  RotationAngleUnits=rad  RotationStandardAxis=+Z  RotationAngle=smiData.RigidTransform(10).angle  RotationArbitraryAxis=smiData.RigidTransform(10).axis  FollAlignAxisA=+X  BaseAlignAxisA=+Y  FollAlignAxisB=+Y  BaseAlignAxisB=+Z  RotationSequenceAxes=FollowerAxes  RotationSequence=XYX  RotationSequenceAngles=[0 0 0]  RotationSequenceAnglesUnits=deg  RotationMatrix=[1 0 0; 0 1 0; 0 0 1]
  Rigid Transform5 : sm_lib/Frames and Transforms/Rigid Transform  TranslationMethod=Cartesian  TranslationStandardOffset=0  TranslationLengthUnit=mm  TranslationStandardAxis=+Z  TranslationCartesianOffset=smiData.RigidTransform(7).translation  TranslationROffset=0  TranslationROffsetUnits=m  TranslationZOffset=0  TranslationZOffsetUnits=m  TranslationThetaOffset=0  TranslationThetaOffsetUnits=deg  RotationMethod=ArbitraryAxis  RotationAngleUnits=rad  RotationStandardAxis=+Z  RotationAngle=smiData.RigidTransform(7).angle  RotationArbitraryAxis=smiData.RigidTransform(7).axis  FollAlignAxisA=+X  BaseAlignAxisA=+Y  FollAlignAxisB=+Y  BaseAlignAxisB=+Z  RotationSequenceAxes=FollowerAxes  RotationSequence=XYX  RotationSequenceAngles=[0 0 0]  RotationSequenceAnglesUnits=deg  RotationMatrix=[1 0 0; 0 1 0; 0 0 1]
  F1 : PMIOPort  Side=Right
  F : PMIOPort  Port=2  Side=Left
  connections:
  Reference Frame/RConn1 -- File Solid/RConn1 -- Rigid Transform4/LConn1 -- Rigid Transform5/LConn1
  Rigid Transform5/RConn1 -- F/RConn1
  Rigid Transform4/RConn1 -- F1/RConn1

== matlab function invertedPendolum/Reverse Pendolum/system ==
  data: x input; xdot output size=4; u input; y output; brake input
function [xdot,y] = pendoloNotLinSys(x,u,brake)
%PENDOLONOTLINSYS Summary of this function goes here
% xDot1:= q2 acc    [rad/s^2]
% xDot2:= q2 vel    [rad/s]
% xDot3:= q1 acc    [rad/s^2]
% xDot4:= q1 vel    [rad/s]

% x1:= q2 dot    [rad/s]
% x2:= q2        [rad]
% x3:= q1 dot    [rad/s]
% x4:= q1        [rad]

% u:= Coppia motore [g/s^2 * mm]
% brake:= true change D2 and shutdown u

coder.extrinsic('evalin', 'assignin')

D1 = 0;                  % Needed in order to set variable class correctly
D1 = evalin('base','D1'); % Read value from workspace

Id = 0;                  % Needed in order to set variable class correctly
Id = evalin('base','Id'); % Read value from workspace

Ibtot = 0;                  % Needed in order to set variable class correctly
Ibtot = evalin('base','Ibtot'); % Read value from workspace

Kmgl = 0;                  % Needed in order to set variable class correctly
Kmgl = evalin('base','Kmgl'); % Read value from workspace

tauMotMax = 0;
tauMotMax = evalin('base','tauMotMax'); % Read value from workspace

rhoInd = 0;                  % Needed in order to set variable class correctly
rhoInd = evalin('base','rhoInd'); % Read value from workspace

rhoMec = 0;                  % Needed in order to set variable class correctly
rhoMec = evalin('base','rhoMec'); % Read value from workspace

D2 = 0;                  % Needed in order to set variable class correctly
D2 = evalin('base','D2'); % Read value from workspace

attDyn = 0;                  % Needed in order to set variable class correctly
attDyn = evalin('base','attDyn'); % Read value from workspace


% Calcoli notevoli:
% fprintf('Kmgl= %f, Ibtot=%f\t', Kmgl, Ibtot); 
skmgl = (Kmgl/Ibtot)*sin(x(4));
% fprintf('skmgl= %f\t', skmgl); 
d1friz = (D1*x(3))/Ibtot;
% fprintf('d1friz= %f\t', d1friz); 
% d2x1 = D2*x(1);
% D2 è in funzione di u, v e si ottiene moltiplicando per l'inerzia i dati
% sperimentali
duty=abs(u/tauMotMax);
if(abs(x(1))>0.001)
%     d2x1 = (((rhoInd)*abs(u/tauMotMax)+ rhoMec)*x(1) + sign(x(1))*attDyn)*Id;
    d2x1 = ((rhoInd+rhoMec)*x(1))*Id + sign(x(1))*attDyn;
%     d2x1 = ((rhoInd*duty+rhoMec)*x(1))*Id + sign(x(1))*attDyn;

else
    d2x1 = 0;

end
% fprintf('d2x1= %f\tduty=%f\n', d2x1,duty); 

xdot=zeros(4,1);
xdot(1) = -(1/Ibtot+1/Id)*d2x1 - skmgl + d1friz + (1/Ibtot+1/Id)*u;
xdot(2) = x(1);
xdot(3) = d2x1/Ibtot + skmgl - d1friz - u/Ibtot;
% fprintf('xdot(3)= %f\n', xdot(3));  
xdot(4) = x(3);


%per ora supponiamo di poter osservare tutto il sistema
y=x;

end

== matlab function invertedPendolum/Reverse Pendolum/saturation ==
  data: x input; xSat output; reset output
function [xSat,reset]  = phisicReaction(x)
%PHISICREACTION Summary of this function goes here
% Funzione che letto lo stato, in caso di urto con la base cambia
% in maniera realistica lo stato introducendo una saturazione.

% xDot1:= q2 acc    [rad/s^2]
% xDot2:= q2 vel    [rad/s]
% xDot3:= q1 acc    [rad/s^2]
% xDot4:= q1 vel    [rad/s]

% x1:= q2 dot    [rad/s]
% x2:= q2        [rad]
% x3:= q1 dot    [rad/s]
% x4:= q1        [rad]

coder.extrinsic('evalin', 'assignin')
q1Max = 0;                  % Needed in order to set variable class correctly
q1Max = evalin('base','q1Max'); % Read value from workspace

xSat=x;
if((abs(x(4))>q1Max)&&(sign(x(3))==sign(x(4))))
    xSat(3)=-x(3)*0.1;          % dissipazione di energia
    xSat(4)=sign(x(4))*(q1Max*0.99999);   % riposizionamento
    
    %to reset integrator state
    assignin('base','x0',xSat); % Assign value back to workspace
    reset=1;
else
    reset=0;
end

end

== matlab function invertedPendolum/Reverse Pendolum/x0Loader ==
  data: x0 output
function x0 = loadX0()
% xDot1:= q2 acc    [rad/s^2]
% xDot2:= q2 vel    [rad/s]
% xDot3:= q1 acc    [rad/s^2]
% xDot4:= q1 vel    [rad/s]

% x1:= q2 dot    [rad/s]
% x2:= q2        [rad]
% x3:= q1 dot    [rad/s]
% x4:= q1        [rad]
coder.extrinsic('evalin', 'assignin')
x0 = zeros(4,1);          % Needed in order to set variable class correctly
x0 = evalin('base','x0'); % Read value from workspace

== matlab function invertedPendolum/Reverse Pendolum/x0Loader1 ==
  data: x0 output
function x0 = loadX0()
% xDot1:= q2 acc    [rad/s^2]
% xDot2:= q2 vel    [rad/s]
% xDot3:= q1 acc    [rad/s^2]
% xDot4:= q1 vel    [rad/s]

% x1:= q2 dot    [rad/s]
% x2:= q2        [rad]
% x3:= q1 dot    [rad/s]
% x4:= q1        [rad]
coder.extrinsic('evalin', 'assignin')
x0 = zeros(4,1);          % Needed in order to set variable class correctly
x0 = evalin('base','x0'); % Read value from workspace

== matlab function invertedPendolum/MATLAB Function ==
  data: mTotDes input; x input; tauMot output size=1
function tauMot = Mwant(mTotDes, x)
% x1:= q2 dot    [rad/s]
% x2:= q2        [rad]
% x3:= q1 dot    [rad/s]
% x4:= q1        [rad]
% tauMot:= Coppia motore [g/s^2 * mm]

coder.extrinsic('evalin', 'assignin')
Kmgl = 0;                  % Needed in order to set variable class correctly
Kmgl = evalin('base','Kmgl'); % Read value from workspace

D1 = 0;                  % Needed in order to set variable class correctly
D1 = evalin('base','D1'); % Read value from workspace

% D2 = 0;                  % Needed in order to set variable class correctly
% D2 = evalin('base','D2'); % Read value from workspace

tauMotMax = 0;           % Needed in order to set variable class correctly
tauMotMax = evalin('base','tauMotMax'); % Read value from workspace

Id = 0;                  % Needed in order to set variable class correctly
Id = evalin('base','Id'); % Read value from workspace


rhoInd = 0;                  % Needed in order to set variable class correctly
rhoInd = evalin('base','rhoInd'); % Read value from workspace

rhoMec = 0;                  % Needed in order to set variable class correctly
rhoMec = evalin('base','rhoMec'); % Read value from workspace

attDyn = 0;                  % Needed in order to set variable class correctly
attDyn = evalin('base','attDyn'); % Read value from workspace

% Frenata del motore in funzione della velocità
% d2x1 = (((rhoInd) *abs(u/tauMotMax) + rhoMec)*x(1) + sign(x(1))*uDym)*Id;

% d2x1 = (((rhoInd) + rhoMec)*x(1) + sign(x(1))*uDym)*Id;
% duty=abs(u/tauMotMax);
if(abs(x(1))>0.001)
%     d2x1 = (((rhoInd)*abs(u/tauMotMax)+ rhoMec)*x(1) + sign(x(1))*attDyn)*Id;
    d2x1 = ((rhoInd+rhoMec)*x(1))*Id + sign(x(1))*attDyn;
%     d2x1 = ((rhoInd*duty+rhoMec)*x(1))*Id + sign(x(1))*attDyn;

else
    d2x1 = 0;

end

% fprintf("d2x1=%f\n",d2x1);

tauMot = -mTotDes + d2x1 + Kmgl*sin(x(4)) - D1*x(3);
% fprintf("tauMot=%f\n",tauMot);
end
